simulink model "Vehicle_Control"  (R2024b)
settings: Solver=ode4  StartTime=0.0  StopTime=20  FixedStep=0.05  RelTol=1e-3
values from neighbouring files (symbols this model uses):
  A = 2.2    [init_vehicle_control.m]
  a_aeb_full = -6.0    (= -6)    [init_vehicle_control.m]
  a_aeb_normal = a_max    (= 2)    [init_vehicle_control.m]
  a_aeb_partial = -3.0    (= -3)    [init_vehicle_control.m]
  a_aeb_warning = a_max    (= 2)    [init_vehicle_control.m]
  a_cmd_test = 0.0    (= 0)    [init_vehicle_control.m]
  a_emergency = -6.0    (= -6)    [init_vehicle_control.m]
  a_max = 2.0    (= 2)    [init_vehicle_control.m]
  a_min = -3.0    (= -3)    [init_vehicle_control.m]
  Cd = 0.30    (= 0.3)    [init_vehicle_control.m]
  Crr = 0.015    [init_vehicle_control.m]
  d0 = 5.0    (= 5)    [init_vehicle_control.m]
  d_full = 15.0    (= 15)    [init_vehicle_control.m]
  d_full_release = 20.0    (= 20)    [init_vehicle_control.m]
  g = 9.81    [init_vehicle_control.m]
  Ki_cruise = 0.15    [init_vehicle_control.m]
  Kp_acc = 0.08    [init_vehicle_control.m]
  Kp_cruise = 0.80    (= 0.8)    [init_vehicle_control.m]
  Kv_acc = 0.40    (= 0.4)    [init_vehicle_control.m]
  m = 1600    [init_vehicle_control.m]
  rho = 1.225    [init_vehicle_control.m]
  T_gap = 1.8    [init_vehicle_control.m]
  TTC_full = 2.0    (= 2)    [init_vehicle_control.m]
  TTC_full_release = 3.0    (= 3)    [init_vehicle_control.m]
  TTC_partial = 3.0    (= 3)    [init_vehicle_control.m]
  TTC_partial_release = 4.0    (= 4)    [init_vehicle_control.m]
  TTC_warning = 4.0    (= 4)    [init_vehicle_control.m]
  TTC_warning_release = 5.0    (= 5)    [init_vehicle_control.m]
  v_ego0 = 20    [init_vehicle_control.m]
  v_set = 25.0    (= 25)    [init_vehicle_control.m]
  x_ego0 = 0    [init_vehicle_control.m]
  x_target0 = 45    [init_vehicle_control.m]
settings Model: Creator=jun_mac  LastModifiedBy=jun_mac

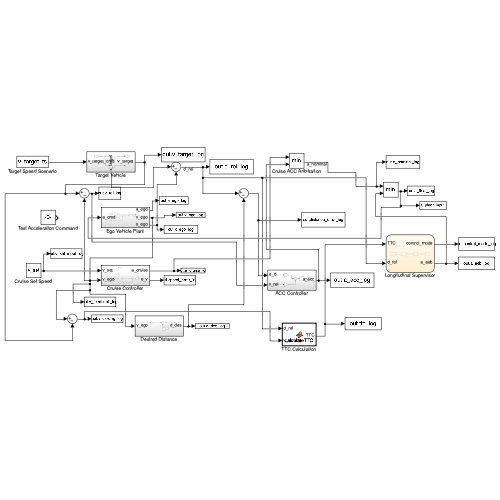
[thumbnail: Simulink's stored preview of the top-level diagram]
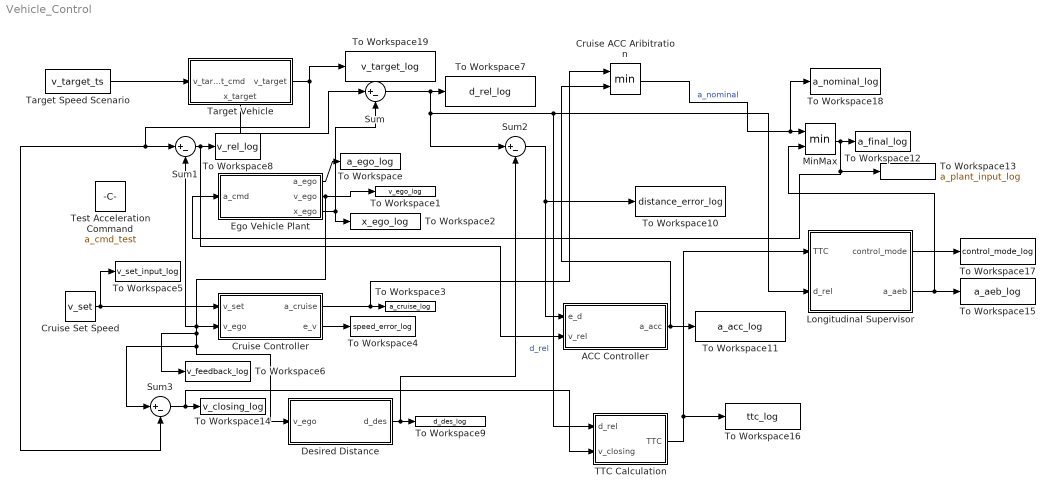
== system Vehicle_Control ==
  ACC Controller : Subsystem
  Cruise ACC Aribitration : MinMax  Inputs=2
  Cruise Controller : Subsystem
  Cruise Set Speed : Constant  Value=v_set
  Desired Distance : Subsystem
  Ego Vehicle Plant : Subsystem
  Longitudinal Supervisor : Stateflow chart  TreatAsAtomicUnit=on
  MinMax : MinMax  Inputs=2
  Sum{,1..3} (4 alike) : Sum  Inputs=|+-
  TTC Calculation : MATLAB Function  TreatAsAtomicUnit=on
  Target Speed Scenario : FromWorkspace  VariableName=v_target_ts
  Target Vehicle : Subsystem
      settings: PortSchema="{\"entries\":[{\"content\":{\"sides\":[{\"content\":{\"connectorIds\":[\"In1\"]},\"type\":\"ConnectorPlacement.EquallySpacedRectSide\",\"uuid\":\"53f13d46-99d8-4fe0-afaf-3d180e73534f\"},{\"content\":{\"connectorIds\":[\"Out1\"],\"side\":\"RIGHT\"},\"type\":\"ConnectorPlacement.EquallySpacedRectSide\",\"uuid\":\"94562ed2-9ba5-4c72-bb5b-571114ff165e\"},{\"content\":{\"side\":\"TOP\"},\"type\":\"ConnectorPlacement.EquallySpacedRectSide\",\"uuid\":\"3fa92fa1-0e7e-48cd-9adb-9803033fd404\"},{\"content\":{\"connectorIds\":[\"Out2\"],\"side\":\"BOTTOM\"},\"type\":\"ConnectorPlacement.EquallySpacedRectSide\",\"uuid\":\"9c73077e-c856-4f4f-abdc-4b6b811b881c\"}]},\"type\":\"ConnectorPlacement.EquallySpacedConnector\",\"uuid\":\"7efa212d-09f3-43c1-915b-6f243c7d1a3c\"}],\"packageUris\":[\"http://schema.mathworks.com/mf0/Connector/R2020b\"],\"version\":\"1.0\"}"
  Test Acceleration Command : Constant  Value=a_cmd_test
  To Workspace : ToWorkspace  VariableName=a_ego_log  SaveFormat=Timeseries  SampleTime=-1
  To Workspace1 : ToWorkspace  VariableName=v_ego_log  SaveFormat=Timeseries  SampleTime=-1
  To Workspace10 : ToWorkspace  VariableName=distance_error_log  SaveFormat=Timeseries  SampleTime=-1
  To Workspace11 : ToWorkspace  VariableName=a_acc_log  SaveFormat=Timeseries  SampleTime=-1
  To Workspace12 : ToWorkspace  VariableName=a_final_log  SaveFormat=Timeseries  SampleTime=-1
  To Workspace13 : ToWorkspace  VariableName=a_plant_input_log  SaveFormat=Timeseries  SampleTime=-1
  To Workspace14 : ToWorkspace  VariableName=v_closing_log  SaveFormat=Timeseries  SampleTime=-1
  To Workspace15 : ToWorkspace  VariableName=a_aeb_log  SaveFormat=Timeseries  SampleTime=-1
  To Workspace16 : ToWorkspace  VariableName=ttc_log  SaveFormat=Timeseries  SampleTime=-1
  To Workspace17 : ToWorkspace  VariableName=control_mode_log  SaveFormat=Timeseries  SampleTime=-1
  To Workspace18 : ToWorkspace  VariableName=a_nominal_log  SaveFormat=Timeseries  SampleTime=-1
  To Workspace19 : ToWorkspace  VariableName=v_target_log  SaveFormat=Timeseries  SampleTime=-1
  To Workspace2 : ToWorkspace  VariableName=x_ego_log  SaveFormat=Timeseries  SampleTime=-1
  To Workspace3 : ToWorkspace  VariableName=a_cruise_log  SaveFormat=Timeseries  SampleTime=-1
  To Workspace4 : ToWorkspace  VariableName=speed_error_log  SaveFormat=Timeseries  SampleTime=-1
  To Workspace5 : ToWorkspace  VariableName=v_set_input_log  SaveFormat=Timeseries  SampleTime=-1
  To Workspace6 : ToWorkspace  VariableName=v_feedback_log  SaveFormat=Timeseries  SampleTime=-1
  To Workspace7 : ToWorkspace  VariableName=d_rel_log  SaveFormat=Timeseries  SampleTime=-1
  To Workspace8 : ToWorkspace  VariableName=v_rel_log  SaveFormat=Timeseries  SampleTime=-1
  To Workspace9 : ToWorkspace  VariableName=d_des_log  SaveFormat=Timeseries  SampleTime=-1
  wires:
  Ego Vehicle Plant/1(a_ego) -> To Workspace/1
  Ego Vehicle Plant/2(v_ego) -> Sum3/1, Desired Distance/1(v_ego), To Workspace6/1, Sum1/2, Cruise Controller/2(v_ego), To Workspace1/1
  Ego Vehicle Plant/3(x_ego) -> Sum/2, To Workspace2/1
  Cruise Controller/1(a_cruise) -> Cruise ACC Aribitration/1, To Workspace3/1
  Cruise Controller/2(e_v) -> To Workspace4/1
  Cruise Set Speed/1 -> Cruise Controller/1(v_set), To Workspace5/1
  Target Speed Scenario/1 -> Target Vehicle/1(v_target_cmd)
  Target Vehicle/2(x_target) -> Sum/1
  Sum/1 -> Longitudinal Supervisor/2(d_rel), TTC Calculation/1(d_rel), Sum2/1, To Workspace7/1  "d_rel"
  Sum1/1 -> ACC Controller/2(v_rel), To Workspace8/1
  Desired Distance/1(d_des) -> Sum2/2, To Workspace9/1
  ACC Controller/1(a_acc) -> Cruise ACC Aribitration/2, To Workspace11/1
  Sum2/1 -> To Workspace10/1, ACC Controller/1(e_d)
  Cruise ACC Aribitration/1 -> To Workspace18/1, MinMax/1  "a_nominal"
  Target Vehicle/1(v_target) -> To Workspace19/1, Sum1/1, Sum3/2
  Sum3/1 -> TTC Calculation/2(v_closing), To Workspace14/1
  TTC Calculation/1(TTC) -> To Workspace16/1, Longitudinal Supervisor/1(TTC)
  Longitudinal Supervisor/1(control_mode) -> To Workspace17/1
  Longitudinal Supervisor/2(a_aeb) -> To Workspace15/1, MinMax/2
  MinMax/1 -> Ego Vehicle Plant/1(a_cmd), To Workspace13/1, To Workspace12/1

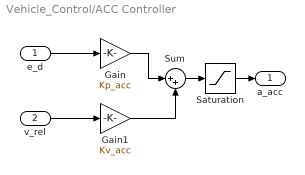
== system Vehicle_Control/ACC Controller ==
  e_d : Inport
  v_rel : Inport  Port=2
  Gain : Gain  Gain=Kp_acc
  Gain1 : Gain  Gain=Kv_acc
  Saturation : Saturate  UpperLimit=a_max  LowerLimit=a_min
  Sum : Sum  Inputs=|++
  a_acc : Outport
  wires:
  v_rel/1 -> Gain1/1
  e_d/1 -> Gain/1
  Gain/1 -> Sum/1
  Gain1/1 -> Sum/2
  Sum/1 -> Saturation/1
  Saturation/1 -> a_acc/1

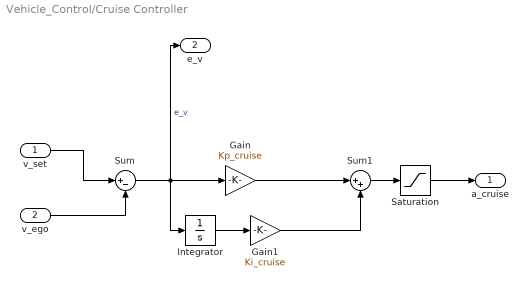
== system Vehicle_Control/Cruise Controller ==
  v_set : Inport
  v_ego : Inport  Port=2
  Gain : Gain  Gain=Kp_cruise
  Gain1 : Gain  Gain=Ki_cruise
  Integrator : Integrator
  Saturation : Saturate  UpperLimit=a_max  LowerLimit=a_min
  Sum : Sum  Inputs=|+-
  Sum1 : Sum  Inputs=|++
  a_cruise : Outport
  e_v : Outport  Port=2
  wires:
  v_set/1 -> Sum/1
  v_ego/1 -> Sum/2
  Sum/1 -> Integrator/1, Gain/1, e_v/1  "e_v"
  Integrator/1 -> Gain1/1
  Gain/1 -> Sum1/1
  Gain1/1 -> Sum1/2
  Sum1/1 -> Saturation/1
  Saturation/1 -> a_cruise/1

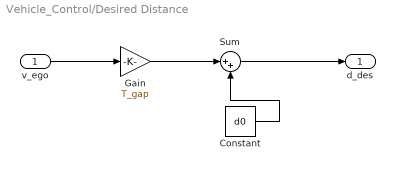
== system Vehicle_Control/Desired Distance ==
  v_ego : Inport
  Constant : Constant  Value=d0
  Gain : Gain  Gain=T_gap
  Sum : Sum  Inputs=|++
  d_des : Outport
  wires:
  v_ego/1 -> Gain/1
  Gain/1 -> Sum/1
  Constant/1 -> Sum/2
  Sum/1 -> d_des/1

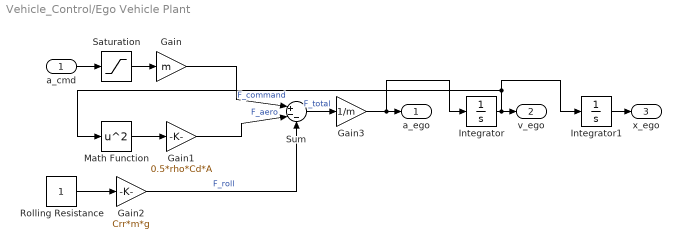
== system Vehicle_Control/Ego Vehicle Plant ==
  a_cmd : Inport
  Gain : Gain  Gain=m
  Gain1 : Gain  Gain=0.5*rho*Cd*A
  Gain2 : Gain  Gain=Crr*m*g
  Gain3 : Gain  Gain=1/m
  Integrator : Integrator  InitialCondition=v_ego0  LimitOutput=on  UpperSaturationLimit=60  LowerSaturationLimit=0
  Integrator1 : Integrator  InitialCondition=x_ego0
  Math Function : Math  Operator=square
  Rolling Resistance : Constant
  Saturation : Saturate  UpperLimit=a_max  LowerLimit=a_emergency
  Sum : Sum  Inputs=|+--
  a_ego : Outport
  v_ego : Outport  Port=2
  x_ego : Outport  Port=3
  wires:
  a_cmd/1 -> Saturation/1
  Saturation/1 -> Gain/1
  Math Function/1 -> Gain1/1
  Gain1/1 -> Sum/2  "F_aero"
  Gain/1 -> Sum/1  "F_command"
  Rolling Resistance/1 -> Gain2/1
  Gain2/1 -> Sum/3  "F_roll"
  Sum/1 -> Gain3/1  "F_total"
  Gain3/1 -> Integrator/1, a_ego/1
  Integrator/1 -> Math Function/1, Integrator1/1, v_ego/1
  Integrator1/1 -> x_ego/1

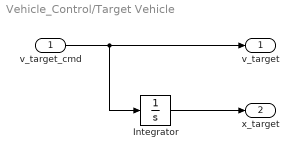
== system Vehicle_Control/Target Vehicle ==
  v_target_cmd : Inport
  Integrator : Integrator  InitialCondition=x_target0
  v_target : Outport
  x_target : Outport  Port=2
  wires:
  v_target_cmd/1 -> v_target/1, Integrator/1
  Integrator/1 -> x_target/1

== matlab function Vehicle_Control/TTC Calculation ==
  data: d_rel input; TTC output; v_closing input
function TTC = calculateTTC(d_rel, v_closing)
%#codegen

if d_rel <= 0

    TTC = 0;

elseif v_closing > 0.1

    TTC = d_rel / v_closing;

else

    TTC = 99;

end

== stateflow chart Vehicle_Control/Longitudinal Supervisor ==
  settings: updateMethod=DISCRETE  sampleTime=Ts
  state NORMAL
    during:
    control_mode = 1;
    a_aeb = a_aeb_normal;
  state AEB_WARNING
    during:
    control_mode = 2;
    a_aeb = a_aeb_warning;
  state AEB_PARTIAL
    during:
    control_mode = 3;
    a_aeb = a_aeb_partial;
  state AEB_FULL
    during:
    control_mode = 4;
    a_aeb = a_aeb_full;
  (default) -> NORMAL
  AEB_WARNING -> NORMAL [order 3] : [TTC >= TTC_warning_release]
  AEB_WARNING -> AEB_PARTIAL [order 2] : [TTC <= TTC_partial]
  AEB_PARTIAL -> AEB_FULL [order 1] : [TTC <= TTC_full || d_rel <= d_full]
  AEB_WARNING -> AEB_FULL [order 1] : [TTC <= TTC_full || d_rel <= d_full]
  NORMAL -> AEB_PARTIAL [order 2] : [TTC <= TTC_partial]
  NORMAL -> AEB_FULL [order 1] : [TTC <= TTC_full || d_rel <= d_full]
  NORMAL -> AEB_WARNING [order 3] : [TTC <= TTC_warning]
  AEB_PARTIAL -> AEB_WARNING [order 2] : [TTC >= TTC_partial_release]
  AEB_FULL -> AEB_PARTIAL : [TTC >= TTC_full_release && d_rel >= d_full_release]
  data: TTC input double size=1; d_rel input double size=1; control_mode output double size=1; a_aeb output double size=1 =a_aeb_normal; TTC_partial parameter double size=1; TTC_full parameter double size=1; TTC_warning parameter double size=1; d_full parameter double size=1; a_aeb_partial parameter double size=1; a_aeb_full parameter double size=1; TTC_warning_release parameter double size=1; TTC_partial_release parameter double size=1; TTC_full_release parameter double size=1; d_full_release parameter double size=1; a_aeb_warning parameter double size=1; a_aeb_normal parameter double size=1
